simulink model "mppt_power_generation_calculation"  (R2024a)
settings: Solver=VariableStepAuto  StartTime=0.0  StopTime=10.0  RelTol=1e-3
undefined symbols (not defined in the file or in its folder): solardata
libraries: spsSeriesRLCBranchLib x2, spsPWMGeneratorDCDCLib x1, spsMosfetLib x1, spsPVArrayLib x1, sps_lib x1
settings Model: Creator=Kshitij Shetty  LastModifiedBy=Kshitij Shetty

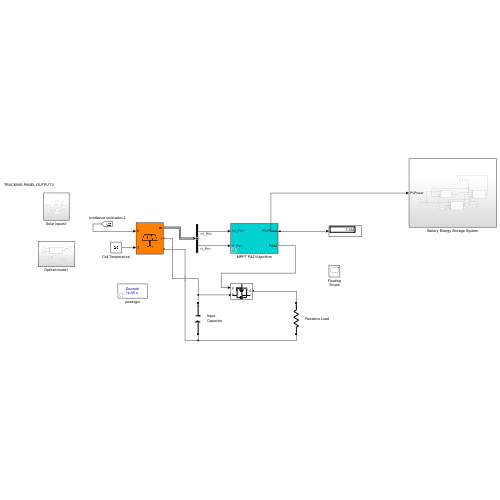
[thumbnail: Simulink's stored preview of the top-level diagram]
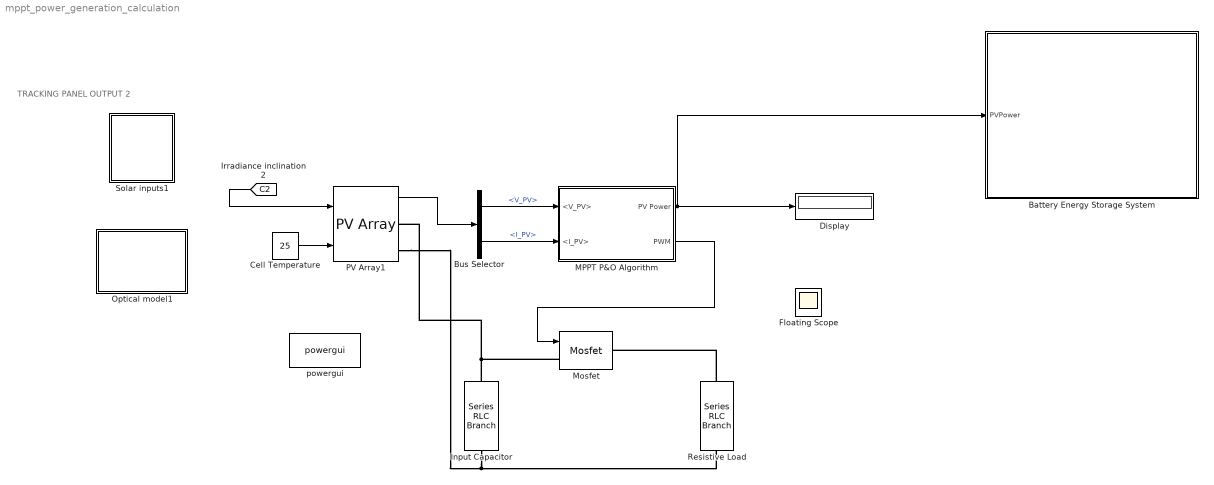
== system mppt_power_generation_calculation ==
  note: TRACKING PANEL OUTPUT 2
  Battery Energy Storage System : Subsystem
  Bus Selector : BusSelector  OutputSignals=V_PV,I_PV
  Cell Temperature : Constant  Value=25
  Display : Display
  Floating Scope : Scope
      settings: Floating=on
  Input Capacitor : spsSeriesRLCBranchLib/Series RLC Branch  LConnTagsString=__new0  RConnTagsString=__new0  BranchType=C  Resistance=10  Inductance=1e-3  SetiL0=off  InitialCurrent=0  Capacitance=1000e-6  Setx0=off  InitialVoltage=0  Measurements=None
  MPPT P&O Algorithm : Subsystem  mask(MPPT Perturb and Observe Algorithm Block){Fsw=1000, StepSize=1e-6}
      mask prompts: Fsw "PWM Switching frequency (Hz):"; StepSize "PWM Duty Cycle (delta) Step Size"
      mask help:
      | MPPT Perturb & Observe Algorithm Block
      | Developed by Rodney Tan (PhD)
      | Version 1.00 Sep 2019
      |
      | This block perform photovoltaic panel Maximum Power Point Tracking based on Perturb & Observe algorithm.
      | This MPPT P&O method is implemented using basic Simulink block only.
      | This MPPT block take in Voltage and Current from photovoltaic panel and output PWM switching signal to drive the DC converter
      mask Help:
      | <b><u>Block Setting</u></b>
      | <b>PWM Switching Frequency (Hz)</b>
      | Specify the PWM switching frequency in Hz.
      | 
      | <b>PWM Duty Cycle Step Size</b>
      | Specify the PWM duty cycle (delta) step size. Default value is 1e-6.
      mask TypeOptions Fsw:
      | PWM Generator
      | (DC-DC)/Fsw
  Mosfet : spsMosfetLib/Mosfet  Ron=0.1  Lon=0  Rd=0.01  Vfd=0  IC=0  Rs=1e5  Cs=inf  Measurements=off
  Optical model1 : Subsystem
  PV Array1 : spsPVArrayLib/PV Array  Npar=1  Nser=4  PlotType=array @ 1000 W/m2 & specified temperatures  S_vec="[ 1000  500  100 ]"  Temp_C_vec="[ 45 25  ]"  ModuleName=User-defined  PlotWhenSelected=off  Pm=250.205  Ncell=60  Voc=37.3  Isc=8.66  Vm=30.7  Im=8.15  beta_Voc_pc=-0.36901  alpha_Isc_pc=0.086998  beta_Voc=-0.13764  alpha_Isc=0.007534  IL=8.7062  I0=4.1579e-10  nI=1.0189  Rsh=240.6015  Rs=0.23732  RobustModel=off  RobustCellTemperature=25  BAL=on  Tc=1e-6  Tfilter=5e-5
  Resistive Load : spsSeriesRLCBranchLib/Series RLC Branch  LConnTagsString=__new0  RConnTagsString=__new0  BranchType=R  Resistance=5  Inductance=1e-3  SetiL0=off  InitialCurrent=0  Capacitance=1e-6  Setx0=off  InitialVoltage=0  Measurements=None
  Solar inputs1 : Subsystem
  powergui : sps_lib/powergui  Priority=1  SimulationMode=Discrete  SampleTime=1e-5  frequency=60  Iterations=50  frequencyindice=0  Pbase=100e6  ErrMax=1e-4  UnitsV=kV  UnitsW=MW  buscounter=0  FunctionMessages=off  echomessages=off  EnableUseOfTLC=off  CurrentSourceSwitches=off  DisableSnubberDevices=off  DisableRonSwitches=off  DisableVfSwitches=off  DisplayEquations=off  AutomaticDiscreteSolvers=off  SolverType=Tustin/Backward Euler (TBE)  Interpol=off  ExternalGateDelay=off  methode=off  Ts=100  x0status=blocks  SPID=off  SwTol=0  HookPort=off  NonlinearTolerance=1e-4  nMaxIteration=100  ContinueOnMaxIteration=off  RestoreLinks=warning  ResistiveCurrentMeasurement=off  Frange=[0:2:500]  Ylog=off  Xlog=on  ShowGrid=off  save=off  variable=ZData  structure=0  ZoomFFT=off  StartTime=0.0  cycles=1  DisplayStyle=1  fundamental=60  FreqAxis=off  MaxFrequency=1000  frequencyindicesteady=1  RmsSteady=1  display=off
  wires:
  MPPT P&O Algorithm/2(PWM) -> Mosfet/1
  Cell Temperature/1 -> PV Array1/2
  MPPT P&O Algorithm/1(PV Power) -> Battery Energy Storage System/1(PVPower), Display/1
  Bus Selector/2 -> MPPT P&O Algorithm/2(<I_PV>)  "<I_PV>"
  PV Array1/1 -> Bus Selector/1
  Bus Selector/1 -> MPPT P&O Algorithm/1(<V_PV>)  "<V_PV>"
  [C2] -> PV Array1/1
  connections:
  PV Array1/RConn2 -- Resistive Load/RConn1 -- Input Capacitor/RConn1
  PV Array1/RConn1 -- Mosfet/LConn1 -- Input Capacitor/LConn1
  Resistive Load/LConn1 -- Mosfet/RConn1

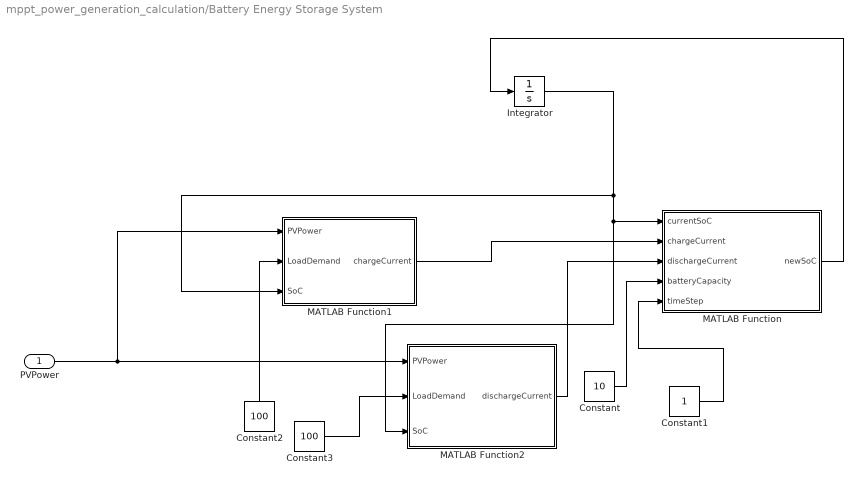
== system mppt_power_generation_calculation/Battery Energy Storage System ==
  PVPower : Inport
  Constant : Constant  Value=10
  Constant1 : Constant
  Constant2 : Constant  Value=100
  Constant3 : Constant  Value=100
  Integrator : Integrator  InitialCondition=0.5
  MATLAB Function : MATLAB Function  TreatAsAtomicUnit=on
  MATLAB Function1 : MATLAB Function  TreatAsAtomicUnit=on
  MATLAB Function2 : MATLAB Function  TreatAsAtomicUnit=on
  wires:
  Constant2/1 -> MATLAB Function1/2(LoadDemand)
  Constant/1 -> MATLAB Function/4(batteryCapacity)
  Constant3/1 -> MATLAB Function2/2(LoadDemand)
  Constant1/1 -> MATLAB Function/5(timeStep)
  Integrator/1 -> MATLAB Function1/3(SoC), MATLAB Function2/3(SoC), MATLAB Function/1(currentSoC)
  MATLAB Function2/1(dischargeCurrent) -> MATLAB Function/3(dischargeCurrent)
  MATLAB Function/1(newSoC) -> Integrator/1
  MATLAB Function1/1(chargeCurrent) -> MATLAB Function/2(chargeCurrent)
  PVPower/1 -> MATLAB Function2/1(PVPower), MATLAB Function1/1(PVPower)

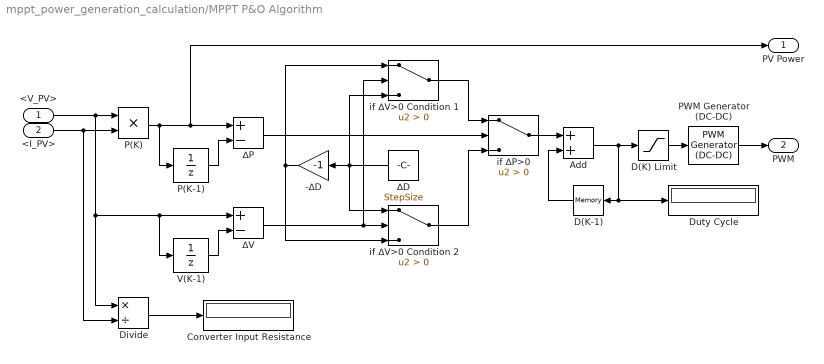
== system mppt_power_generation_calculation/MPPT P&O Algorithm ==
  <V_PV> : Inport
  <I_PV> : Inport  Port=2
  -∆D : Gain  Gain=-1
  Add : Sum
  Converter Input Resistance : Display
  D(K) Limit : Saturate  UpperLimit=1  LowerLimit=0
  D(K-1) : Memory  InitialCondition=0.5  InheritSampleTime=on
  Divide : Product  Inputs=*/
  Duty Cycle : Display
  P(K) : Product
  P(K-1) : UnitDelay  SampleTime=-1  HasFrameUpgradeWarning=on
  PWM Generator (DC-DC) : spsPWMGeneratorDCDCLib/PWM Generator (DC-DC)  Fsw=Fsw  Ts=0
  V(K-1) : UnitDelay  SampleTime=-1  HasFrameUpgradeWarning=on
  if ∆P>0 : Switch  Criteria=u2 > Threshold  SaturateOnIntegerOverflow=off  InputSameDT=off
  if ∆V>0 Condition 1 : Switch  Criteria=u2 > Threshold  SaturateOnIntegerOverflow=off  InputSameDT=off
  if ∆V>0 Condition 2 : Switch  Criteria=u2 > Threshold  SaturateOnIntegerOverflow=off  InputSameDT=off
  ∆D : Constant  Value=StepSize
  ∆P : Sum  Inputs=+-
  ∆V : Sum  Inputs=+-
  PV Power : Outport  VectorParamsAs1DForOutWhenUnconnected=off
  PWM : Outport  Port=2  VectorParamsAs1DForOutWhenUnconnected=off
  wires:
  P(K)/1 -> ∆P/1, PV Power/1, P(K-1)/1
  <I_PV>/1 -> P(K)/2, Divide/2
  if ∆P>0/1 -> Add/1
  if ∆V>0 Condition 1/1 -> if ∆P>0/1
  ∆P/1 -> if ∆P>0/2
  P(K-1)/1 -> ∆P/2
  V(K-1)/1 -> ∆V/2
  ∆V/1 -> if ∆V>0 Condition 2/2, if ∆V>0 Condition 1/2
  <V_PV>/1 -> Divide/1, ∆V/1, V(K-1)/1, P(K)/1
  Add/1 -> D(K) Limit/1, Duty Cycle/1, D(K-1)/1
  if ∆V>0 Condition 2/1 -> if ∆P>0/3
  D(K-1)/1 -> Add/2
  ∆D/1 -> if ∆V>0 Condition 2/1, -∆D/1, if ∆V>0 Condition 1/3
  -∆D/1 -> if ∆V>0 Condition 2/3, if ∆V>0 Condition 1/1
  PWM Generator (DC-DC)/1 -> PWM/1
  Divide/1 -> Converter Input Resistance/1
  D(K) Limit/1 -> PWM Generator (DC-DC)/1

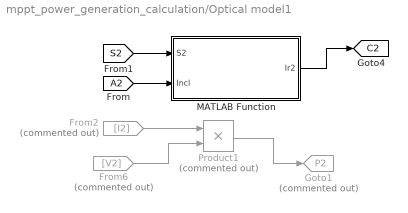
== system mppt_power_generation_calculation/Optical model1 ==
  From2 : From  Commented=on  GotoTag=I2
  From6 : From  Commented=on  GotoTag=V2
  Goto1 : Goto  Commented=on  GotoTag=P2  TagVisibility=global
  MATLAB Function : MATLAB Function  TreatAsAtomicUnit=on
  Product1 : Product  Commented=on
  tag scope: C2=global
  wires:
  MATLAB Function/1(Ir2) -> [C2]
  Product1/1 -> Goto1/1
  From2/1 -> Product1/1
  From6/1 -> Product1/2
  [A2] -> MATLAB Function/2(Incl)
  [S2] -> MATLAB Function/1(S2)

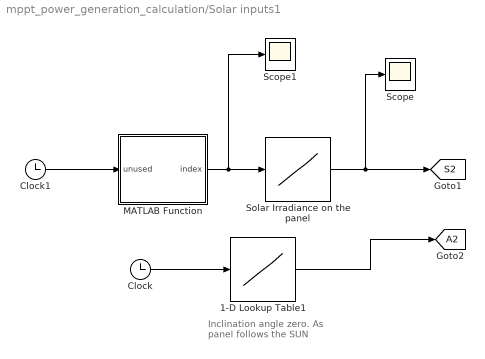
== system mppt_power_generation_calculation/Solar inputs1 ==
  note: Inclination angle zero.
      | As panel follows the SUN
  1-D Lookup Table1 : Lookup_n-D  NumberOfTableDimensions=1  BreakpointsForDimension1=1:721  Table=zeros(1, 721)  InternalRulePriority=Speed  RndMeth=Simplest
  Clock : Clock
  Clock1 : Clock
  MATLAB Function : MATLAB Function  TreatAsAtomicUnit=on
  Scope : Scope
  Scope1 : Scope
  Solar Irradiance on the panel : Lookup_n-D  NumberOfTableDimensions=1  BreakpointsForDimension1=1:length(solardata)  Table=solardata  InternalRulePriority=Speed  RndMeth=Simplest
  tag scope: A2=global, S2=global
  wires:
  1-D Lookup Table1/1 -> [A2]
  Clock/1 -> 1-D Lookup Table1/1
  Solar Irradiance on the panel/1 -> Scope/1, [S2]
  Clock1/1 -> MATLAB Function/1(unused)
  MATLAB Function/1(index) -> Scope1/1, Solar Irradiance on the panel/1

== matlab function mppt_power_generation_calculation/Optical model1/MATLAB Function ==
  data: S2 input; Ir2 output; Incl input
function Ir2 = optics2(S2, Incl)
    
    %This function computes the reflection, absorption and transmission in
    %the glass to compute the irradiation to the PV cells, the heat absorbed 
    %in the glass and the radiation power absorbed in the PV cells,
    %it is based on Fresnel's laws, depending on the incident angle
    
    Ncell =  72;
    Acell =  0.0225;
    ng = 1.52;
    absg = 0.2;
    dg = 0.01;
    rpv = 0.15;
   

    % Fresnel equations 1st boundary
    r1p =  ( ng^2*cos(Incl) - sqrt(ng^2 - sin(Incl)^2) )^2/( ng^2*cos(Incl) + sqrt( ng^2 - sin(Incl)^2 ) )^2; %P polarization
    r1s =  ( cos(Incl) - sqrt(ng^2 - sin(Incl)^2) )^2/( cos(Incl) + sqrt( ng^2 - sin(Incl)^2 ) )^2; %S polarization
    r1 = 0.5*(r1p + r1s); %Effective reflectance
    t1 = 1-r1;

    nga = 1/ng; %refractive index glass -> air
    th2 = asin(sin(Incl)/ng);  %Snell's law to compute angle of incidence on 2nd boundary

    % Fresnel equations 2nd boundary
    r2p = ( nga^2*cos(th2) - sqrt(nga^2 - sin(th2)^2) )^2/( nga^2*cos(th2) + sqrt( nga^2 - sin(th2)^2 ) )^2 ;
    r2s = ( cos(th2) - sqrt(nga^2 - sin(th2)^2) )^2/( cos(th2) + sqrt( nga^2 - sin(th2)^2 ) )^2 ;
    r2 = 0.5*(r2p + r2s); %Effective reflectance
    t2 = 1 - r2;

    taug = exp(-absg*dg/cos(th2)); 
    
    %Total coefficients for infinite reflections between 2 parallel boundaries
    Transg = t1*taug*t2/(1 - r1*r2*taug^2);
    Reflg = r1 + (t1^2*taug^2*r2)/(1 - r1*r2*taug^2);
    Absg = 1 - Transg - Reflg; 

    Ir2 = S2*Transg; %Irradiation to the PV cells
    heatg = Acell*Ncell*Absg*S2; %heat absorbed in the glass
    powAbspv = Acell*Ncell*Transg*(1-rpv)*S2; %radiation power absorbed by PV cells. Part of it transforms in electrical power
    
end

== matlab function mppt_power_generation_calculation/Battery Energy Storage System/MATLAB Function ==
  data: currentSoC input; newSoC output; chargeCurrent input; dischargeCurrent input; batteryCapacity input; timeStep input
function newSoC = SoCCalculation(currentSoC, chargeCurrent, dischargeCurrent, batteryCapacity, timeStep)
    % Calculate the new state of charge
    newSoC = currentSoC + (chargeCurrent - dischargeCurrent) * timeStep / batteryCapacity;
    % Limit the SoC between 0 and 1
    newSoC = max(0, min(1, newSoC));
end

== matlab function mppt_power_generation_calculation/Battery Energy Storage System/MATLAB Function1 ==
  data: PVPower input; chargeCurrent output; LoadDemand input; SoC input
function chargeCurrent = chargeControl(PVPower, LoadDemand, SoC)
    maxChargeCurrent = 50; % Maximum charging current in amps
    if SoC < 0.95 % Charge battery if SoC is less than 95%
        excessPower = PVPower - LoadDemand;
        chargeCurrent = min(excessPower / 3.7, maxChargeCurrent); % Adjust based on battery voltage
    else
        chargeCurrent = 0; % Stop charging if SoC >= 95%
    end
end

== matlab function mppt_power_generation_calculation/Battery Energy Storage System/MATLAB Function2 ==
  data: PVPower input; dischargeCurrent output; LoadDemand input; SoC input
function dischargeCurrent = dischargeControl(PVPower, LoadDemand, SoC)
    maxDischargeCurrent = 50; % Maximum discharging current in amps
    if SoC > 0.2 % Discharge battery if SoC is more than 20%
        deficitPower = LoadDemand - PVPower;
        dischargeCurrent = min(deficitPower / 3.7, maxDischargeCurrent); % Adjust based on battery voltage
    else
        dischargeCurrent = 0; 
        % Stop discharging if SoC <= 20%
    end
end

== matlab function mppt_power_generation_calculation/Solar inputs1/MATLAB Function ==
  data: unused input; index output
function index = time_to_index(~)
    datetimeNow = datetime('now');
    [~, ~, ~, hour, minute, ~] = datevec(datetimeNow);
    var_a = hour*60 + minute ;
    index = var_a/2.0 +1 ;
end
